simulink model "three_phase_inv(single)"  (R2023a)
settings: Solver=VariableStepAuto  StartTime=0.0  StopTime=10.0  RelTol=1e-3
libraries: spsIGBTLib x6, simulink x3, spsDCVoltageSourceLib x1, spsGroundLib x1, spsSawtoothGeneratorLib x1, spsThreePhaseParallelRLCBranchLib x1, spsThreePhaseVIMeasurementLib x1, spspowerguiLib x1
settings Model: Creator=jain  LastModifiedBy=banof
settings DebuggingCC: UnconnectedInputMsg=warning  UnconnectedOutputMsg=warning  UnconnectedLineMsg=warning
settings ModelReferenceCC: EnableRefExpFcnMdlSchedulingChecks=on
settings RTWCC: DLArmComputeVersion=19.05

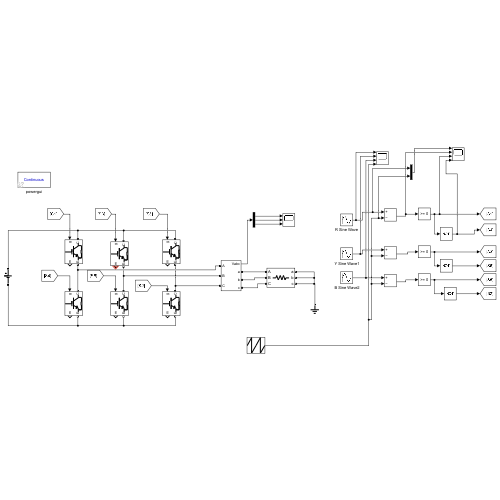
[thumbnail: Simulink's stored preview of the top-level diagram]
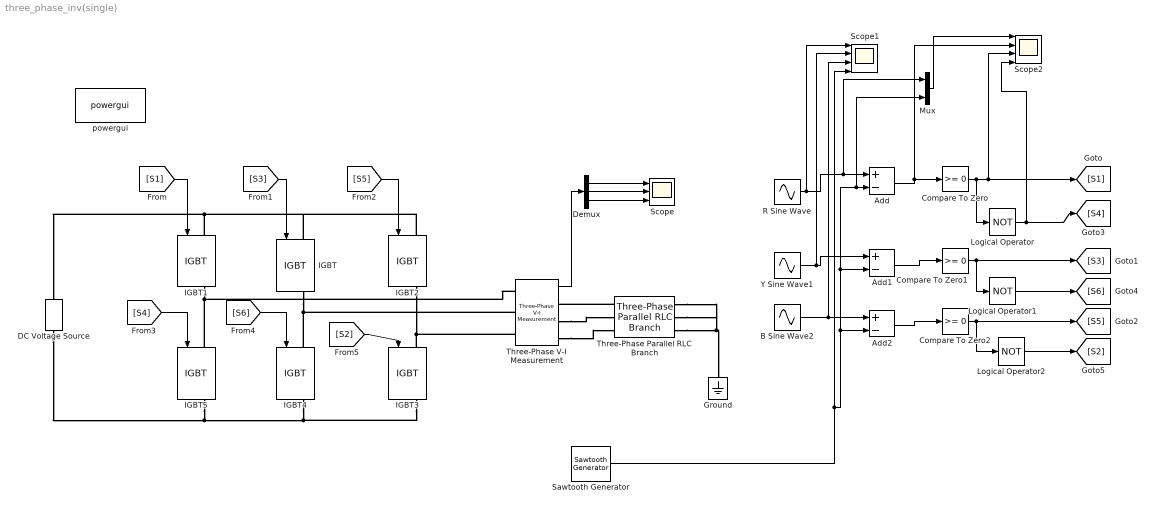
== system three_phase_inv(single) ==
  " B Sine Wave2" : Sin  Frequency=2*pi*50  Phase=-2*pi/3  SampleTime=0
  " Y Sine Wave1" : Sin  Frequency=2*pi*50  Phase=2*pi/3  SampleTime=0
  Add : Sum  Inputs=+-
  Add1 : Sum  Inputs=+-
  Add2 : Sum  Inputs=+-
  Compare To Zero : simulink/Logic and Bit Operations/Compare To Zero  relop=>=  OutDataTypeStr=boolean
  Compare To Zero1 : simulink/Logic and Bit Operations/Compare To Zero  relop=>=  OutDataTypeStr=boolean
  Compare To Zero2 : simulink/Logic and Bit Operations/Compare To Zero  relop=>=  OutDataTypeStr=boolean
  DC Voltage Source : spsDCVoltageSourceLib/DC Voltage Source  Amplitude=100  Measurements=None
  Demux : Demux  Outputs=3
  Ground : spsGroundLib/Ground  LConnTagsString=a
  IGBT{,1..5} (6 alike) : spsIGBTLib/IGBT  Ron=0.001  Lon=0  Vf=1  Tf=1e-6  Tt=2e-6  IC=0  Rs=1e5  Cs=inf  Measurements=on
  Logical Operator : Logic  Operator=NOT  Inputs=1  AllPortsSameDT=off  OutDataTypeStr=boolean
  Logical Operator1 : Logic  Operator=NOT  Inputs=1  AllPortsSameDT=off  OutDataTypeStr=boolean
  Logical Operator2 : Logic  Operator=NOT  Inputs=1  AllPortsSameDT=off  OutDataTypeStr=boolean
  Mux : Mux  Inputs=2
  R Sine Wave : Sin  Frequency=2*pi*50  SampleTime=0
  Sawtooth Generator : spsSawtoothGeneratorLib/Sawtooth Generator  Freq=1e3  Phase=180  Ts=0
  Scope : Scope  NumInputPorts=3
  Scope1 : Scope  NumInputPorts=4
  Scope2 : Scope  NumInputPorts=4
  Three-Phase Parallel RLC Branch : spsThreePhaseParallelRLCBranchLib/Three-Phase Parallel RLC Branch  LConnTagsString=A|B|C  RConnTagsString=A|B|C  BranchType=R  Resistance=1  Inductance=1e-3  Capacitance=1e-6  Measurements=None
  Three-Phase V-I Measurement : spsThreePhaseVIMeasurementLib/Three-Phase V-I Measurement  VoltageMeasurement=phase-to-phase  SetLabelV=off  LabelV=Vabc  Vpu=off  VpuLL=off  CurrentMeasurement=no  SetLabelI=off  LabelI=Iabc  Ipu=off  Pbase=100e6  Vbase=500e3  OutputType=Complex  PhasorSimulation=off  PSBequivalent=0
  powergui : spspowerguiLib/powergui  Priority=1  SimulationMode=Continuous  SampleTime=50e-6  frequency=60  Iterations=50  frequencyindice=0  Pbase=100e6  ErrMax=1e-4  UnitsV=kV  UnitsW=MW  buscounter=0  FunctionMessages=off  echomessages=off  EnableUseOfTLC=off  CurrentSourceSwitches=off  DisableSnubberDevices=off  DisableRonSwitches=off  DisableVfSwitches=off  DisplayEquations=off  AutomaticDiscreteSolvers=off  SolverType=Tustin/Backward Euler (TBE)  Interpol=off  ExternalGateDelay=off  methode=off  Ts=100  x0status=blocks  SPID=on  SwTol=0  HookPort=off  NonlinearTolerance=1e-4  nMaxIteration=100  ContinueOnMaxIteration=off  RestoreLinks=warning  ResistiveCurrentMeasurement=off  Frange=[0:2:500]  Ylog=off  Xlog=on  ShowGrid=off  save=off  variable=ZData  structure=0  ZoomFFT=off  StartTime=0.0  cycles=1  DisplayStyle=1  fundamental=60  FreqAxis=off  MaxFrequency=1000  frequencyindicesteady=1  RmsSteady=1  display=off
  wires:
  Sawtooth Generator/1 -> Scope1/4, Add2/2, Add1/2, Mux/2, Add/2
  R Sine Wave/1 -> Scope1/1, Mux/1, Add/1
  " Y Sine Wave1"/1 -> Scope1/2, Add1/1
  " B Sine Wave2"/1 -> Scope1/3, Add2/1
  Add2/1 -> Compare To Zero2/1
  Add1/1 -> Compare To Zero1/1
  Add/1 -> Scope2/2, Compare To Zero/1
  Compare To Zero/1 -> Logical Operator/1, Scope2/3, [S1]
  Compare To Zero1/1 -> Logical Operator1/1, [S3]
  Compare To Zero2/1 -> Logical Operator2/1, [S5]
  Logical Operator/1 -> [S4], Scope2/4
  Logical Operator1/1 -> [S6]
  Logical Operator2/1 -> [S2]
  [S4] -> IGBT5/1
  [S6] -> IGBT4/1
  [S2] -> IGBT3/1
  [S5] -> IGBT2/1
  [S3] -> IGBT/1
  [S1] -> IGBT1/1
  Demux/1 -> Scope/1
  Demux/2 -> Scope/2
  Demux/3 -> Scope/3
  Three-Phase V-I Measurement/1 -> Demux/1
  Mux/1 -> Scope2/1
  connections:
  Three-Phase V-I Measurement/LConn1 -- IGBT5/LConn1 -- IGBT1/RConn1
  Three-Phase V-I Measurement/LConn2 -- IGBT/RConn1 -- IGBT4/LConn1
  Three-Phase V-I Measurement/LConn3 -- IGBT3/LConn1 -- IGBT2/RConn1
  IGBT2/LConn1 -- IGBT/LConn1 -- IGBT1/LConn1 -- DC Voltage Source/RConn1
  DC Voltage Source/LConn1 -- IGBT5/RConn1 -- IGBT4/RConn1 -- IGBT3/RConn1
  Three-Phase Parallel RLC Branch/LConn1 -- Three-Phase V-I Measurement/RConn1
  Three-Phase V-I Measurement/RConn2 -- Three-Phase Parallel RLC Branch/LConn2
  Three-Phase V-I Measurement/RConn3 -- Three-Phase Parallel RLC Branch/LConn3
  Three-Phase Parallel RLC Branch/RConn3 -- Three-Phase Parallel RLC Branch/RConn1 -- Three-Phase Parallel RLC Branch/RConn2 -- Ground/LConn1
